simulink model "linearizedModel_withObs"  (R2022b)
settings: Solver=VariableStepAuto  StartTime=0.0  StopTime=30  RelTol=1e-3
values from neighbouring files (symbols this model uses):
  A = zeros(6,6)    [sim1_PartD.m]    (also in sim2_PartF.m; sim3_partG_part1.m; sim4_partG_part2.m)
  B = [0,1/M,0,-1/M/l1,0,-1/M/l2]'    [sim1_PartD.m]    (also in sim2_PartF.m)
  C = zeros(3,6)    [sim1_PartD.m]    (also in sim2_PartF.m = [1,0,0,0,0,0; sim3_partG_part1.m = CC(var_sel,:); sim4_partG_part2.m = CC(var_sel,:))
  D = zeros(3,1)    [sim1_PartD.m]    (also in sim2_PartF.m = zeros(size(C,1),1); sim3_partG_part1.m = zeros(n_output_var,1); sim4_partG_part2.m = zeros(n_output_var,1))
  init_state = [x0,xd0,theta1_0,theta1_d0,theta2_0,theta2_d0]'    [sim1_PartD.m]    (also in sim2_PartF.m = [5,-0.5,20/180*pi,-0.5,-20/180*pi,0.5]'; sim3_partG_part1.m = [5,-0.5,20/180*pi,-0.5,-20/180*pi,0.5]'; sim4_partG_part2.m = [0,0,0,0,0,0]')
  L = LT'    [sim2_PartF.m]    (also in sim3_partG_part1.m = P*C'*sigma_v_inv; sim4_partG_part2.m = P*C'*sigma_v_inv)
  u_gain = 100    [sim2_PartF.m]
  var_sel = [1,3,5]    [sim2_PartF.m]    (also in sim3_partG_part1.m; sim4_partG_part2.m)
settings Model: Creator=liuji  LastModifiedBy=liuji

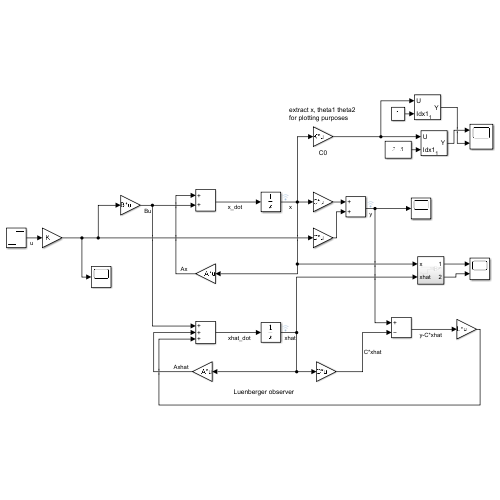
[thumbnail: Simulink's stored preview of the top-level diagram]
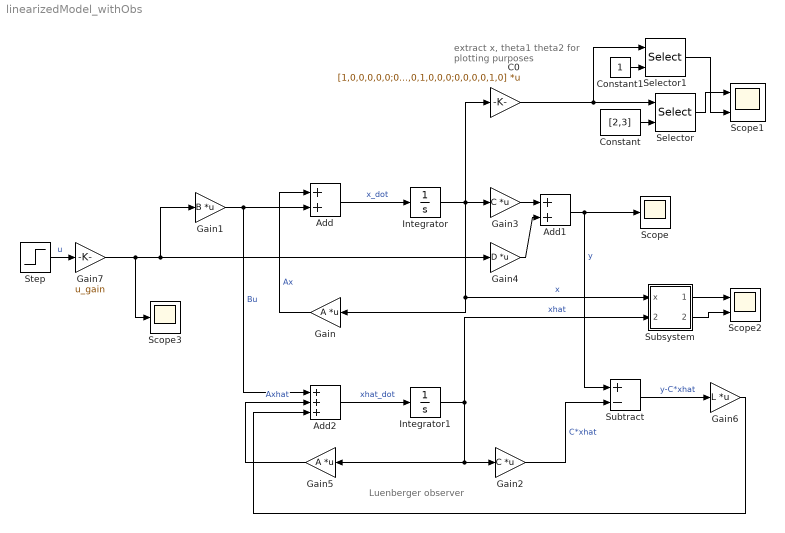
== system linearizedModel_withObs ==
  note: Luenberger observer
  note: extract x, theta1 theta2
      | for plotting purposes
  Add : Sum
  Add1 : Sum
  Add2 : Sum  Inputs=+++
  C0 : Gain  Gain=[1,0,0,0,0,0;0,0,1,0,0,0;0,0,0,0,1,0]  Multiplication=Matrix(K*u)
  Constant : Constant  Value=[2,3]
  Constant1 : Constant
  Gain : Gain  Gain=A  Multiplication=Matrix(K*u)
  Gain1 : Gain  Gain=B  Multiplication=Matrix(K*u)
  Gain2 : Gain  Gain=C  Multiplication=Matrix(K*u)
  Gain3 : Gain  Gain=C  Multiplication=Matrix(K*u)
  Gain4 : Gain  Gain=D  Multiplication=Matrix(K*u)
  Gain5 : Gain  Gain=A  Multiplication=Matrix(K*u)
  Gain6 : Gain  Gain=L  Multiplication=Matrix(K*u)
  Gain7 : Gain  Gain=u_gain
  Integrator : Integrator  InitialCondition=init_state
  Integrator1 : Integrator  InitialCondition=[0,0,0,0,0,0]'
  Scope : Scope
  Scope1 : Scope  NumInputPorts=2
  Scope2 : Scope  NumInputPorts=2
  Scope3 : Scope
  Selector : Selector  InputPortWidth=3  IndexOptions=Index vector (port)  Indices=[1 3]  OutputSizes=1
  Selector1 : Selector  InputPortWidth=3  IndexOptions=Index vector (port)  Indices=[1 3]  OutputSizes=1
  Step : Step  Time=0  SampleTime=0
  Subsystem : Subsystem
  Subtract : Sum  Inputs=+-
  wires:
  Integrator/1 -> Gain3/1, C0/1, Subsystem/1(x), Gain/1  "x"
  Add/1 -> Integrator/1  "x_dot"
  Gain/1 -> Add/1  "Ax"
  Gain3/1 -> Add1/1
  Gain4/1 -> Add1/2
  Constant/1 -> Selector/2
  Selector/1 -> Scope1/1
  Constant1/1 -> Selector1/2
  Selector1/1 -> Scope1/2
  Gain1/1 -> Add2/1, Add/2  "Bu"
  C0/1 -> Selector1/1, Selector/1
  Add1/1 -> Scope/1, Subtract/1  "y"
  Integrator1/1 -> Subsystem/2(xhat), Gain2/1, Gain5/1  "xhat"
  Add2/1 -> Integrator1/1  "xhat_dot"
  Gain5/1 -> Add2/2  "Axhat"
  Step/1 -> Gain7/1  "u"
  Gain2/1 -> Subtract/2  "C*xhat"
  Subtract/1 -> Gain6/1  "y-C*xhat"
  Gain6/1 -> Add2/3
  Subsystem/1(Out1) -> Scope2/1
  Subsystem/2(Out2) -> Scope2/2
  Gain7/1 -> Scope3/1, Gain4/1, Gain1/1

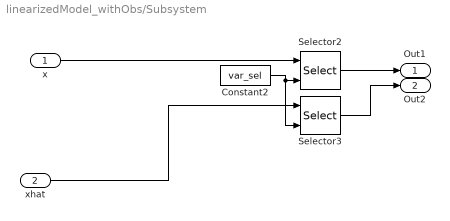
== system linearizedModel_withObs/Subsystem ==
  x : Inport
  xhat : Inport  Port=2
  Constant2 : Constant  Value=var_sel
  Selector2 : Selector  InputPortWidth=6  IndexOptions=Index vector (port)  Indices=[1 3]  OutputSizes=1
  Selector3 : Selector  InputPortWidth=6  IndexOptions=Index vector (port)  Indices=[1 3]  OutputSizes=1
  Out1 : Outport
  Out2 : Outport  Port=2
  wires:
  xhat/1 -> Selector3/1
  Constant2/1 -> Selector3/2, Selector2/2
  Selector2/1 -> Out1/1
  x/1 -> Selector2/1
  Selector3/1 -> Out2/1
